simulink model "sgMdl_IO135_DMALoopback"  (R2024b)
settings: Solver=FixedStepAuto  StartTime=0.0  StopTime=inf  RelTol=1e-3  EnableMultiTasking=on
libraries: speedgoatlib_IO135 x3, speedgoatlib_interrupt x1, dspsrcs4 x1
Description:
  | IO135 - DMA Loopback
settings Model: sg_rtwmakecfg_data=_sglibc_  ModifiedByFormat=Speedgoat  Creator=Speedgoat  LastModifiedBy=Speedgoat
settings SolverCC: ConcurrentTasks=on  AlgebraicLoopSolver=TrustRegion  PositivePriorityOrder=on  AutoInsertRateTranBlk=on  InsertRTBMode=Never (minimum delay)
settings DataIOCC: SaveFormat=StructureWithTime  ReturnWorkspaceOutputs=off
settings OptimizationCC: BlockReduction=off  OptimizeBlockIOStorage=off  BufferReuse=off  GlobalBufferReuse=off  ExpressionFolding=off  LocalBlockOutputs=off
settings DebuggingCC: TasksWithSamePriorityMsg=none  UnconnectedInputMsg=warning  UnconnectedOutputMsg=warning  UnconnectedLineMsg=warning  SFExecutionAtInitializationDiag=none  ArithmeticOperatorsInVariantConditions=warning
settings HardwareCC: ProdBitPerLong=64  ProdLongLongMode=on  ProdHWDeviceType=Intel->x86-64 (Linux 64)
settings ModelReferenceCC: EnableRefExpFcnMdlSchedulingChecks=on
settings SFSimCC: SimUseLocalCustomCode=off  CustomCodeUndefinedFunction=UseInterfaceOnly
settings RTWCC: Description=Speedgoat Real-Time Target Machine  SystemTargetFile=speedgoat.tlc  TemplateMakefile=slrealtime_default_tmf  PostCodeGenCommand=sg.model.build.makeCfg(bdroot, buildInfo);  RTWUseLocalCustomCode=off  Toolchain=Simulink Real-Time Toolchain  BuildConfiguration=Faster Runs  TargetLang=C++  GPUComputeCapability=3.5  DLArmComputeVersion=19.05
settings CodeAppCC: StateflowObjectComments=on
settings SimulinkRealTimeTargetCC: SubcomponentCodeInterfacePackaging=Reusable function  InstructionSetFMA=off  LogToMDFFile=off  SLRTFileLogMaxRuns=10  UseGCCFastMath=on
settings ConfigComp: CovBoundaryAbsTol=1.0e-5

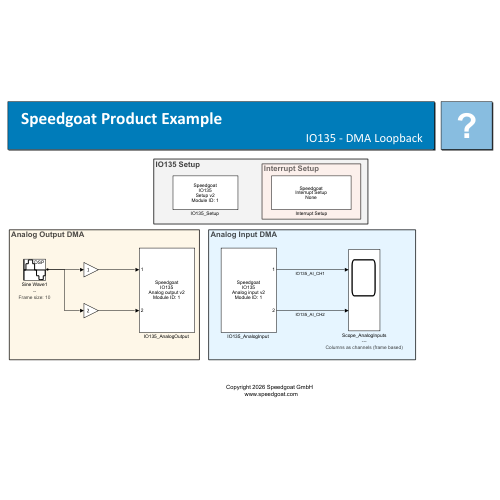
[thumbnail: Simulink's stored preview of the top-level diagram]
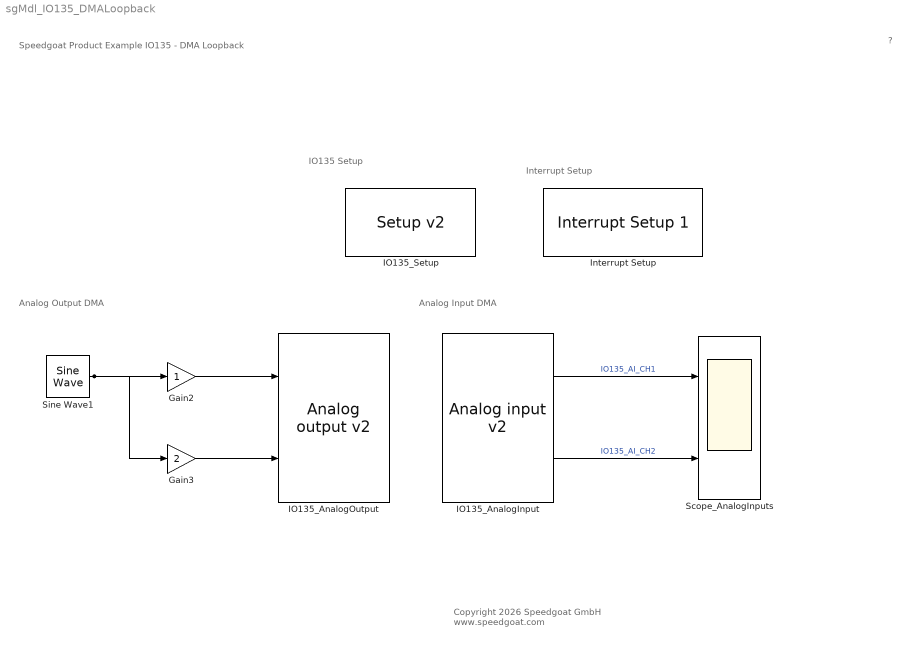
== system sgMdl_IO135_DMALoopback ==
  note: Interrupt Setup
  note: IO135 Setup
  note: Analog Input DMA
  note: Analog Output DMA
  note: Speedgoat Product Example
      | IO135 - DMA Loopback
  note: ?
  note: Copyright 2026 Speedgoat GmbH
      |  www.speedgoat.com
  Gain2 : Gain
  Gain3 : Gain  Gain=2
  "IO135_AnalogInput " : speedgoatlib_IO135/Analog input v2   parModuleId=1  parSampleTime=-1  parPciSlot=-1  parAdcChannels=[1 2]  parAdcVoltageRange=[2 2 2 2]  parAdcOversamplRate=[1 1 1 1]  parAdcContSampling=0  parAdcDmaEnable=1  parAdcActiveDmaDevices=[1 1 1 1]  parAdcFrameSize=10
      settings: SourceProductName=Simulink Real-Time: Speedgoat I/O Driver Library
  "IO135_AnalogOutput " : speedgoatlib_IO135/Analog output v2   parModuleId=1  parSampleTime=-1  parPciSlot=-1  parDacChannels=[1 2]  parDacVoltageRange=[5 5 5 5 5 5 5 5 5 5 5 5 5 5 5 5]  parDacInitValues=[0 0]  parDacReset=[1 1]  parDacSyncOut=1  parDacDmaEnable=1  parDacActiveDmaDevices=[1 1 1 1]  parDacDmaLatency=2  parDacFrameSize=10
      settings: SourceProductName=Simulink Real-Time: Speedgoat I/O Driver Library
  "IO135_Setup " : speedgoatlib_IO135/Setup v2   parPciSlot=-1  parModuleId=1  parInterModuleSync=None  parConvClockBaseRate=20MHz  parConvClock1Divider=2000  parConvClock2Divider=2000  parFrameTriggerEnable=on  parFrameTriggerDivider=10  parConvClock1BaseRate=1  parConvClock2BaseRate=1  parFrameTriggerClock=1  parAdcChannels=[1 2]  parAdcRange1=+-10V  parAdcRange2=+-10V  parAdcRange3=+-10V  parAdcRange4=+-10V  parAdcVoltageRange=[2 2 2 2]  parAdcOversampling1=None  parAdcOversampling2=None  parAdcOversampling3=None  parAdcOversampling4=None  parAdcOversamplRate=[1 1 1 1]  parAdcContSampling=off  parAdcDataCorrection=Automatic  parAdcCorrectionActive={}  parAdcCorrectionPm5V={'1','0','0';'2','0','0';'3','0','0';'4','0','0';'5','0','0';'6','0','0';'7','0','0';'8','0','0';'9','0','0';'10','0','0';'11','0','0';'12','0','0';'13','0','0';'14','0',' 0';'15','0','0';'16','0','0';'17','0','0';'18','0','0';'19','0','0';'20','0','0';'21','0','0';'22','0','0';'23','0','0';'24','0','0';'25','0','0';'26','0','0';'27','0','0';'28','0','0';'29','0','0';'30','0','0';'31','0','0';'32','0','0'}  parAdcCorrectionPm10V={'1','0','0';'2','0','0';'3','0','0';'4','0','0';'5','0','0';'6','0','0';'7','0','0';'8','0','0';'9','0','0';'10','0','0';'11','0','0';'12','0','0';'13','0','0';'14','0',' 0';'15','0','0';'16','0','0';'17','0','0';'18','0','0';'19','0','0';'20','0','0';'21','0','0';'22','0','0';'23','0','0';'24','0','0';'25','0','0';'26','0','0';'27','0','0';'28','0','0';'29','0','0';'30','0','0';'31','0','0';'32','0','0'}  parAdcDmaEnable=on  parAdcDmaClock=Clock 1  parAdcFrameSize_=10  parAdcSampleTime_=-1  parAdcActiveDmaDevices=[1 1 1 1]  parAdcFrameTriggerEnable=1  parAdcFrameSize=10  parAdcSampleTime=0.001  parDacChannels=[1 2]  parDacInitValues=0  parDacReset=1  parDacRange1=+-10V  parDacRange2=+-10V  parDacRange3=+-10V  parDacRange4=+-10V  parDacRange5=+-10V  parDacRange6=+-10V  parDacRange7=+-10V  parDacRange8=+-10V  parDacRange9=+-10V  parDacRange10=+-10V  parDacRange11=+-10V  parDacRange12=+-10V  parDacRange13=+-10V  parDacRange14=+-10V  parDacRange15=+-10V  parDacRange16=+-10V  parDacVoltageRange=[5 5 5 5 5 5 5 5 5 5 5 5 5 5 5 5]  parDacSyncOut=on  parDacDataCorrection=Automatic  parDacCorrectionActive={}  parDacCorrection5V={'1','0','0';'2','0','0';'3','0','0';'4','0','0';'5','0','0';'6','0','0';'7','0','0';'8','0','0';'9','0','0';'10','0','0';'11','0','0';'12','0','0';'13','0','0';'14','0',' 0';'15','0','0';'16','0','0'}  parDacCorrection10V={'1','0','0';'2','0','0';'3','0','0';'4','0','0';'5','0','0';'6','0','0';'7','0','0';'8','0','0';'9','0','0';'10','0','0';'11','0','0';'12','0','0';'13','0','0';'14','0',' 0';'15','0','0';'16','0','0'}  parDacCorrection10_8V={'1','0','0';'2','0','0';'3','0','0';'4','0','0';'5','0','0';'6','0','0';'7','0','0';'8','0','0';'9','0','0';'10','0','0';'11','0','0';'12','0','0';'13','0','0';'14','0',' 0';'15','0','0';'16','0','0'}  parDacCorrectionPm5V={'1','0','0';'2','0','0';'3','0','0';'4','0','0';'5','0','0';'6','0','0';'7','0','0';'8','0','0';'9','0','0';'10','0','0';'11','0','0';'12','0','0';'13','0','0';'14','0',' 0';'15','0','0';'16','0','0'}  parDacCorrectionPm10V={'1','0','0';'2','0','0';'3','0','0';'4','0','0';'5','0','0';'6','0','0';'7','0','0';'8','0','0';'9','0','0';'10','0','0';'11','0','0';'12','0','0';'13','0','0';'14','0',' 0';'15','0','0';'16','0','0'}  parDacCorrectionPm10_8V={'1','0','0';'2','0','0';'3','0','0';'4','0','0';'5','0','0';'6','0','0';'7','0','0';'8','0','0';'9','0','0';'10','0','0';'11','0','0';'12','0','0';'13','0','0';'14','0',' 0';'15','0','0';'16','0','0'}  parDacDmaEnable=on  parDacDmaLatency=Until next frame  parDacDmaClock=Clock 1  parDacFrameSize_=10  parDacSampleTime_=-1  parDacActiveDmaDevices=[1 1 1 1]  parDacFrameTriggerEnable=1  parDacFrameSize=10  parDacSampleTime=0.001  parDoChannels=1  parDoInitValues=0  parDoReset=1  parDiChannels=5  parDiDebounceEnable=off  parDiDebounceTime=0  parDiDebounceValue=0  parDioPullRefFront=Pull-up 3.3V  parDioPullRefRear=Floating
      settings: SourceProductName=Simulink Real-Time: Speedgoat I/O Driver Library
  Interrupt Setup : speedgoatlib_interrupt/Interrupt Setup 1  parModuleTrigger=on  parPollingMode=off  parPriorityConf=High  parPriority=241  confStartFcn=IO135_start_public  confStopFcn=IO135_stop_public  confIsrFcn=IO135_isr_public  confMapFcn=IO135_map_public  confHookFile=io135_int_hooks.c  confIrqNr=-1  confIsPolling=off  confModID=16776961  confSelectedInt=Speedgoat IO135 DMA interrupt  confSelectedId=1  confSelectedChannel=[]  confData=[]  confForcePollingMode=off
  Scope_AnalogInputs : Scope  NumInputPorts=2
      settings: AttributesFormatString=|
      | ---
      | %<FrameBasedProcessingString>
  Sine Wave1 : dspsrcs4/Sine Wave  Amplitude=1  Frequency=100  Phase=0  SampleMode=Discrete  OutComplex=Real  CompMethod=Trigonometric fcn  TableSize=Speed  SampleTime=1/10000  SamplesPerFrame=10  ResetState=Restart at time zero  OutputFrames=off  dataType=double  wordLen=16  udDataType=sfix(16)  fracBitsMode=Best precision  numFracBits=15  OutDataTypeStr=double  LastOutDataTypeStr=double
      settings: AttributesFormatString=|
      | --
      | Frame size: %<SamplesPerFrame>
  wires:
  Sine Wave1/1 -> Gain2/1, Gain3/1
  "IO135_AnalogInput "/1 -> Scope_AnalogInputs/1  "IO135_AI_CH1"
  Gain2/1 -> "IO135_AnalogOutput "/1
  Gain3/1 -> "IO135_AnalogOutput "/2
  "IO135_AnalogInput "/2 -> Scope_AnalogInputs/2  "IO135_AI_CH2"
